simulink model "Thrust_Direction_quad"  (R2013a)
settings: Solver=ode45  StartTime=0.0  StopTime=10.0  RelTol=1e-3
values from neighbouring files (symbols this model uses):
  g = 9.8    [PID_init.m]    (also in quad_init.m)
  m = 0.835    [PID_init.m]    (also in quad_init.m)
undefined symbols (not defined in the file or in its folder): q_d
libraries: quad_lib x2, aerolibutil x2, aerolibtransform2 x1
settings Model: Creator=diogo  LastModifiedBy=diogo

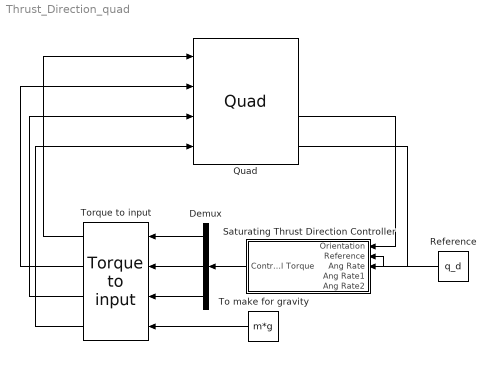
== system Thrust_Direction_quad ==
  Demux : Demux  Outputs=3
  Quad : quad_lib/Quad
  Reference : Constant  Value=q_d
  Saturating Thrust Direction Controller : Subsystem
  To make for gravity : Constant  Value=m*g
  Torque to input : quad_lib/PID_quad/Torque to input
  wires:
  Saturating Thrust Direction Controller/1(Control Torque) -> Demux/1
  Demux/1 -> Torque to input/1
  Demux/2 -> Torque to input/2
  Demux/3 -> Torque to input/3
  Torque to input/4 -> Quad/4
  Torque to input/3 -> Quad/3
  Torque to input/2 -> Quad/2
  Torque to input/1 -> Quad/1
  To make for gravity/1 -> Torque to input/4
  Quad/3 -> Saturating Thrust Direction Controller/1(Orientation)
  Quad/4 -> Saturating Thrust Direction Controller/3(Ang Rate)
  Reference/1 -> Saturating Thrust Direction Controller/2(Reference)

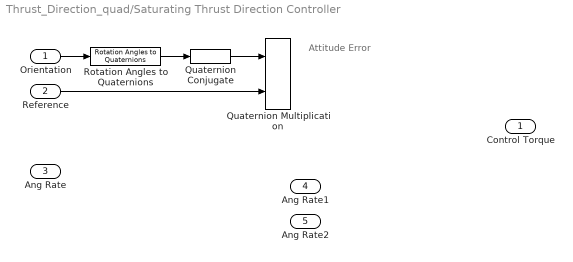
== system Thrust_Direction_quad/Saturating Thrust Direction Controller ==
  note: Attitude Error
  Orientation : Inport
  Reference : Inport  Port=2
  Ang Rate : Inport  Port=3
  Ang Rate1 : Inport  Port=4
  Ang Rate2 : Inport  Port=5
  Quaternion Conjugate : aerolibutil/Quaternion Conjugate
  Quaternion Multiplication : aerolibutil/Quaternion Multiplication
  Rotation Angles to Quaternions : aerolibtransform2/Rotation Angles to Quaternions  rotationOrder=XYZ
  Control Torque : Outport
  wires:
  Orientation/1 -> Rotation Angles to Quaternions/1
  Rotation Angles to Quaternions/1 -> Quaternion Conjugate/1
  Reference/1 -> Quaternion Multiplication/2
  Quaternion Conjugate/1 -> Quaternion Multiplication/1
